simulink model "feedbackLinearization"  (Simulink 7.0)
settings: Solver=ode45  StartTime=0.0  StopTime=10.0  RelTol=1e-3
settings Model: Creator=wizest  LastModifiedBy=wizest

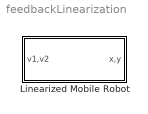
== system feedbackLinearization ==
  Linearized Mobile Robot : Subsystem

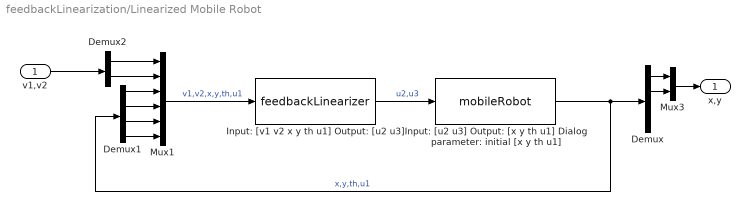
== system feedbackLinearization/Linearized Mobile Robot ==
  v1,v2 : Inport  OutDataType=sfix(16)  OutScaling=2^0
  Demux : Demux
  Demux1 : Demux
  Demux2 : Demux  Outputs=2
  Input: [u2 u3] Output: [x y th u1] Dialog parameter: initial [x y th u1] : M-S-Function  FunctionName=mobileRobot  Parameters=[5 5 1 1]
  Input: [v1 v2 x y th u1] Output: [u2 u3] : M-S-Function  FunctionName=feedbackLinearizer  Parameters=0
  Mux1 : Mux  Inputs=6
  Mux3 : Mux  Inputs=2
  x,y : Outport  OutDataType=sfix(16)  OutScaling=2^0
  wires:
  Demux/1 -> Mux3/1
  Demux/2 -> Mux3/2
  Mux1/1 -> Input: [v1 v2 x y th u1] Output: [u2 u3]/1  "v1,v2,x,y,th,u1"
  Demux1/1 -> Mux1/3
  Demux1/2 -> Mux1/4
  Input: [v1 v2 x y th u1] Output: [u2 u3]/1 -> Input: [u2 u3] Output: [x y th u1] Dialog parameter: initial [x y th u1]/1  "u2,u3"
  Input: [u2 u3] Output: [x y th u1] Dialog parameter: initial [x y th u1]/1 -> Demux/1, Demux1/1  "x,y,th,u1"
  Demux1/3 -> Mux1/5
  Demux1/4 -> Mux1/6
  Demux2/1 -> Mux1/1
  Demux2/2 -> Mux1/2
  v1,v2/1 -> Demux2/1
  Mux3/1 -> x,y/1
